simulink model "BMP388"  (R2020a)
settings: Solver=FixedStepAuto  StartTime=0.0  StopTime=10.0  RelTol=1e-3
values from neighbouring files (symbols this model uses):
  BMP388_pressure_variance = 1.2^2    (= 1.44)    [configure_simulation.m]
  BMP388_sample_rate = 10    [configure_simulation.m]
  BMP388_temperature_variance = 1    [configure_simulation.m]
libraries: simulink x7
settings Model: Creator=Philip  LastModifiedBy=Philip

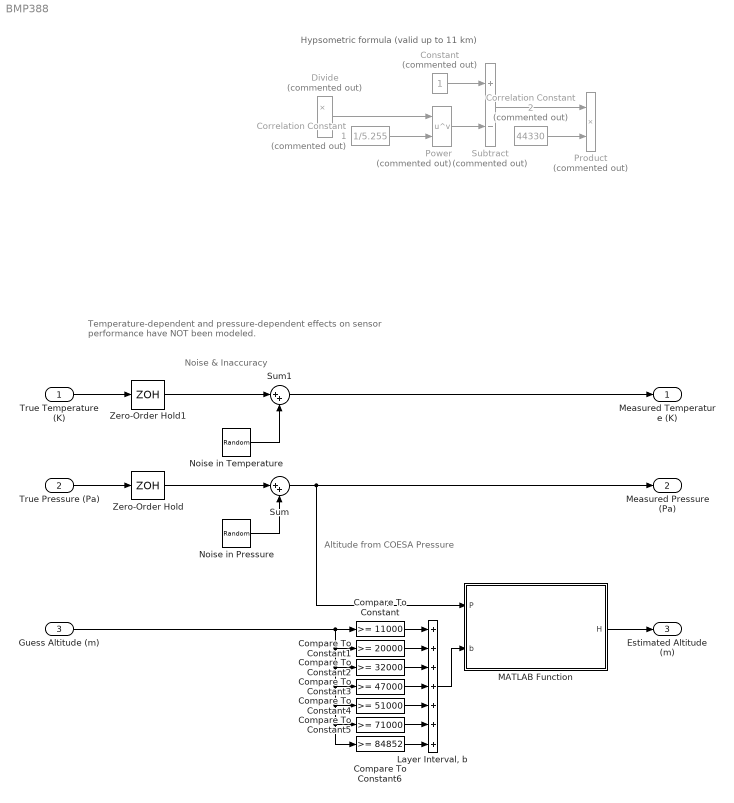
== system BMP388 ==
  note: Altitude from COESA Pressure
  note: Temperature-dependent and pressure-dependent effects on sensor performance have NOT been modeled.
  note: Noise & Inaccuracy
  note: Hypsometric formula (valid up to 11 km)
  True Temperature (K) : Inport
  True Pressure (Pa) : Inport  Port=2
  Guess Altitude (m) : Inport  Port=3
  Compare To Constant : simulink/Logic and Bit Operations/Compare To Constant  relop=>=  const=11000  OutDataTypeStr=uint8
  Compare To Constant1 : simulink/Logic and Bit Operations/Compare To Constant  relop=>=  const=20000  OutDataTypeStr=uint8
  Compare To Constant2 : simulink/Logic and Bit Operations/Compare To Constant  relop=>=  const=32000  OutDataTypeStr=uint8
  Compare To Constant3 : simulink/Logic and Bit Operations/Compare To Constant  relop=>=  const=47000  OutDataTypeStr=uint8
  Compare To Constant4 : simulink/Logic and Bit Operations/Compare To Constant  relop=>=  const=51000  OutDataTypeStr=uint8
  Compare To Constant5 : simulink/Logic and Bit Operations/Compare To Constant  relop=>=  const=71000  OutDataTypeStr=uint8
  Compare To Constant6 : simulink/Logic and Bit Operations/Compare To Constant  relop=>=  const=84852  OutDataTypeStr=uint8
  Constant : Constant  Commented=on
  Correlation Constant 1 : Constant  Commented=on  Value=1/5.255
  Correlation Constant 2 : Constant  Commented=on  Value=44330
  Divide : Product  Commented=on  Inputs=*/
  "Layer Interval, b" : Sum  Inputs=+++++++
  MATLAB Function : MATLAB Function  TreatAsAtomicUnit=on
  Noise in Pressure : RandomNumber  Variance=BMP388_pressure_variance  SampleTime=1/BMP388_sample_rate
  Noise in Temperature : RandomNumber  Variance=BMP388_temperature_variance  SampleTime=1/BMP388_sample_rate
  Power : Math  Commented=on  Operator=pow  SaturateOnIntegerOverflow=on
  Product : Product  Commented=on
  Subtract : Sum  Commented=on  Inputs=+-
  Sum : Sum  Inputs=|++
  Sum1 : Sum  Inputs=|++
  Zero-Order Hold : ZeroOrderHold  SampleTime=1/BMP388_sample_rate
  Zero-Order Hold1 : ZeroOrderHold  SampleTime=1/BMP388_sample_rate
  Measured Temperature (K) : Outport
  Measured Pressure (Pa) : Outport  Port=2
  Estimated Altitude (m) : Outport  Port=3
  wires:
  Correlation Constant 1/1 -> Power/2
  Divide/1 -> Power/1
  Power/1 -> Subtract/2
  Constant/1 -> Subtract/1
  Subtract/1 -> Product/1
  Correlation Constant 2/1 -> Product/2
  True Pressure (Pa)/1 -> Zero-Order Hold/1
  Noise in Pressure/1 -> Sum/2
  Noise in Temperature/1 -> Sum1/2
  True Temperature (K)/1 -> Zero-Order Hold1/1
  Guess Altitude (m)/1 -> Compare To Constant3/1, Compare To Constant4/1, Compare To Constant5/1, Compare To Constant6/1, Compare To Constant2/1, Compare To Constant1/1, Compare To Constant/1
  Compare To Constant/1 -> "Layer Interval, b"/1
  Compare To Constant1/1 -> "Layer Interval, b"/2
  Compare To Constant2/1 -> "Layer Interval, b"/3
  "Layer Interval, b"/1 -> MATLAB Function/2(b)
  Compare To Constant3/1 -> "Layer Interval, b"/4
  Compare To Constant4/1 -> "Layer Interval, b"/5
  Compare To Constant5/1 -> "Layer Interval, b"/6
  Compare To Constant6/1 -> "Layer Interval, b"/7
  MATLAB Function/1(H) -> Estimated Altitude (m)/1
  Sum/1 -> MATLAB Function/1(P), Measured Pressure (Pa)/1
  Sum1/1 -> Measured Temperature (K)/1
  Zero-Order Hold1/1 -> Sum1/1
  Zero-Order Hold/1 -> Sum/1

== matlab function BMP388/MATLAB Function ==
  data: P input; H output; b input
function H = altitude_from_pressure(P, b)
R = 287.053; % [J/kg/K] gas constant (air)
g0 = 9.80665; % [m/s^2] standard gravity

% Hb [km]    geopotential height at base of layer b
% Lb [K/km]  lapse rate across layer b
% Pb [Pa]    static pressure at base of layer b
% Tb [K]     temperature at base of layer b

if b == 0
    Hb = 0; 
    Lb = -6.5e-3;
    Pb = 101325;
    Tb = 288.15;
elseif b == 1
    Hb = 11000; 
    Lb = 0.0;
    Pb = 22632.06;
    Tb = 216.65;
elseif b == 2
    Hb = 20000; 
    Lb = 1.0e-3;
    Pb = 5474.889;
    Tb = 216.65;
elseif b == 3
    Hb = 32000; 
    Lb = 2.8e-3;
    Pb = 868.0187;
    Tb = 228.65;
elseif b == 4
    Hb = 47000; 
    Lb = 0.0;
    Pb = 110.9063;
    Tb = 270.65;
elseif b == 5
    Hb = 51000; 
    Lb = -2.8e-3;
    Pb = 66.93887;
    Tb = 270.65;
elseif b == 6
    Hb = 71000; 
    Lb = -2.0e-3;
    Pb = 3.956420;
    Tb = 288.15;
elseif b == 7
    Hb = 84852; 
    Lb = nan;
    Pb = 0.3734;
    Tb = 186.87;
else
    Hb = nan; 
    Lb = nan;
    Pb = nan;
    Tb = nan; 
end

if isnan(Lb)
    H = nan;
elseif Lb == 0
    H = Hb - log(P/Pb)*R*Tb/g0;
else
    T = Tb * (P/Pb)^(-Lb*R/g0);
    H = Hb + (T - Tb) / Lb;
end
end
